simulink library "INP_BRK_ManOver"  (R2024b)
settings: Solver=VariableStepAuto  StartTime=0.0  StopTime=10.0  RelTol=1e-3
undefined symbols (not defined in the file): INP_BRK_p_PrsBrkFrLoLim_bar, INP_BRK_p_PrsBrkFrMan_bar, INP_BRK_p_PrsBrkFrUpLim_bar, INP_BRK_p_PrsBrkReLoLim_bar, INP_BRK_p_PrsBrkReMan_bar, INP_BRK_p_PrsBrkReUpLim_bar, INP_BRK_p_SwtPrsBrkFrMan_na, INP_BRK_p_SwtPrsBrkReMan_na
libraries: simulink x2
settings Model: Creator=blatak  LastModifiedBy=jmbsp

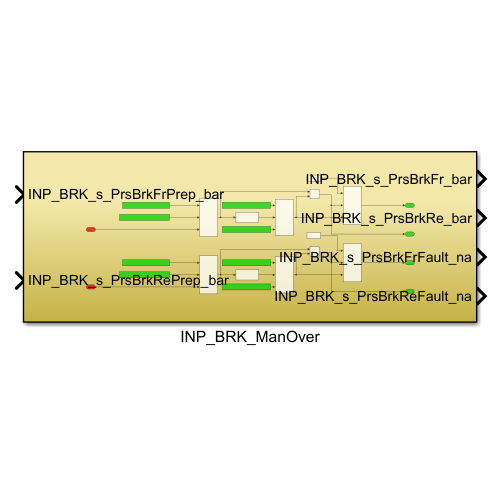
[thumbnail: Simulink's stored preview of the top-level diagram]
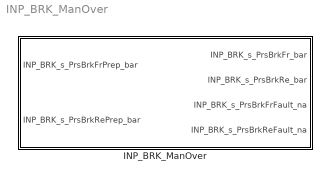
== system INP_BRK_ManOver ==
  INP_BRK_ManOver : Subsystem

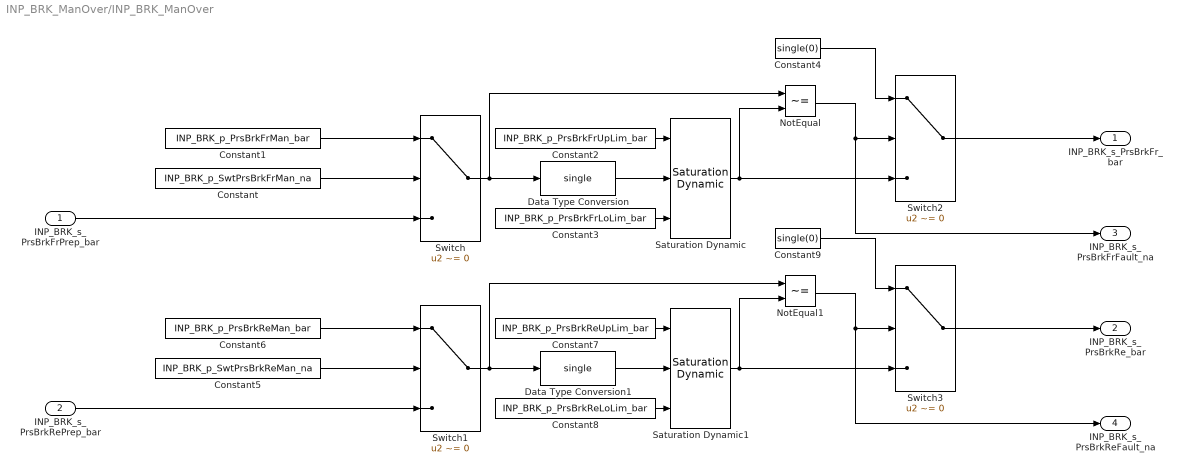
== system INP_BRK_ManOver/INP_BRK_ManOver ==
  INP_BRK_s_PrsBrkFrPrep_bar : Inport
  INP_BRK_s_PrsBrkRePrep_bar : Inport  Port=2
  Constant : Constant  Description=|  Value=INP_BRK_p_SwtPrsBrkFrMan_na
      | Switch for manual override of the longitudinal acceleration value, if 1 instead the measured 
      | value the INP_IMU_p_ALgtVehMan_mps2 is used
  Constant1 : Constant  Description=|  Value=INP_BRK_p_PrsBrkFrMan_bar
      | Value for longitudinal acceleration, which is used if the INP_IMU_p_SwtAXxxVehMan_na
      | is set to 1 instead of the measured value
  Constant2 : Constant  Description=Upper saturation limit for longitudinal acceleration  Value=INP_BRK_p_PrsBrkFrUpLim_bar
  Constant3 : Constant  Description=Lower saturation limit for longitudinal acceleration  Value=INP_BRK_p_PrsBrkFrLoLim_bar
  Constant4 : Constant  Value=single(0)
  Constant5 : Constant  Description=|  Value=INP_BRK_p_SwtPrsBrkReMan_na
      | Switch for manual override of the longitudinal acceleration value, if 1 instead the measured 
      | value the INP_IMU_p_ALgtVehMan_mps2 is used
  Constant6 : Constant  Description=|  Value=INP_BRK_p_PrsBrkReMan_bar
      | Value for longitudinal acceleration, which is used if the INP_IMU_p_SwtAXxxVehMan_na
      | is set to 1 instead of the measured value
  Constant7 : Constant  Description=Upper saturation limit for longitudinal acceleration  Value=INP_BRK_p_PrsBrkReUpLim_bar
  Constant8 : Constant  Description=Lower saturation limit for longitudinal acceleration  Value=INP_BRK_p_PrsBrkReLoLim_bar
  Constant9 : Constant  Value=single(0)
  Data Type Conversion : DataTypeConversion  OutDataTypeStr=single  SaturateOnIntegerOverflow=off  RndMeth=Floor
  Data Type Conversion1 : DataTypeConversion  OutDataTypeStr=single  SaturateOnIntegerOverflow=off  RndMeth=Floor
  NotEqual : RelationalOperator  Operator=~=  OutDataTypeStr=boolean  RndMeth=Simplest  InputSameDT=off
  NotEqual1 : RelationalOperator  Operator=~=  OutDataTypeStr=boolean  RndMeth=Simplest  InputSameDT=off
  Saturation Dynamic : simulink/Discontinuities/Saturation Dynamic  OutMin=[]  OutMax=[]  OutDataTypeStr=Inherit: Same as second input  OutDataType=fixdt(1, 16)  OutScaling=2^-10  DoSatur=off
  Saturation Dynamic1 : simulink/Discontinuities/Saturation Dynamic  OutMin=[]  OutMax=[]  OutDataTypeStr=Inherit: Same as second input  OutDataType=fixdt(1, 16)  OutScaling=2^-10  DoSatur=off
  Switch{,1..3} (4 alike) : Switch  Criteria=u2 ~= 0  SaturateOnIntegerOverflow=off  InputSameDT=off
  INP_BRK_s_PrsBrkFr_bar : Outport
  INP_BRK_s_PrsBrkRe_bar : Outport  Port=2
  INP_BRK_s_PrsBrkFrFault_na : Outport  Port=3
  INP_BRK_s_PrsBrkReFault_na : Outport  Port=4
  wires:
  Switch2/1 -> INP_BRK_s_PrsBrkFr_bar/1
  Constant2/1 -> Saturation Dynamic/1
  Constant4/1 -> Switch2/1
  Constant1/1 -> Switch/1
  Switch/1 -> Data Type Conversion/1, NotEqual/1
  Constant/1 -> Switch/2
  Saturation Dynamic1/1 -> NotEqual1/2, Switch3/3
  Switch1/1 -> Data Type Conversion1/1, NotEqual1/1
  Constant9/1 -> Switch3/1
  Constant3/1 -> Saturation Dynamic/3
  Saturation Dynamic/1 -> NotEqual/2, Switch2/3
  NotEqual/1 -> INP_BRK_s_PrsBrkFrFault_na/1, Switch2/2
  Data Type Conversion/1 -> Saturation Dynamic/2
  Constant6/1 -> Switch1/1
  Constant8/1 -> Saturation Dynamic1/3
  Data Type Conversion1/1 -> Saturation Dynamic1/2
  INP_BRK_s_PrsBrkRePrep_bar/1 -> Switch1/3
  NotEqual1/1 -> INP_BRK_s_PrsBrkReFault_na/1, Switch3/2
  Switch3/1 -> INP_BRK_s_PrsBrkRe_bar/1
  Constant5/1 -> Switch1/2
  Constant7/1 -> Saturation Dynamic1/1
  INP_BRK_s_PrsBrkFrPrep_bar/1 -> Switch/3
